simulink model "EjemploClient"  (Simulink 8.1)
settings: Solver=ode3  StartTime=0.0  StopTime=inf  FixedStep=0.01  RelTol=1e-3
libraries: aerolibanimutils x1
settings Model: Creator=Usuario  LastModifiedBy=emanuel
settings OptimizationCC: SimCompilerOptimization=On

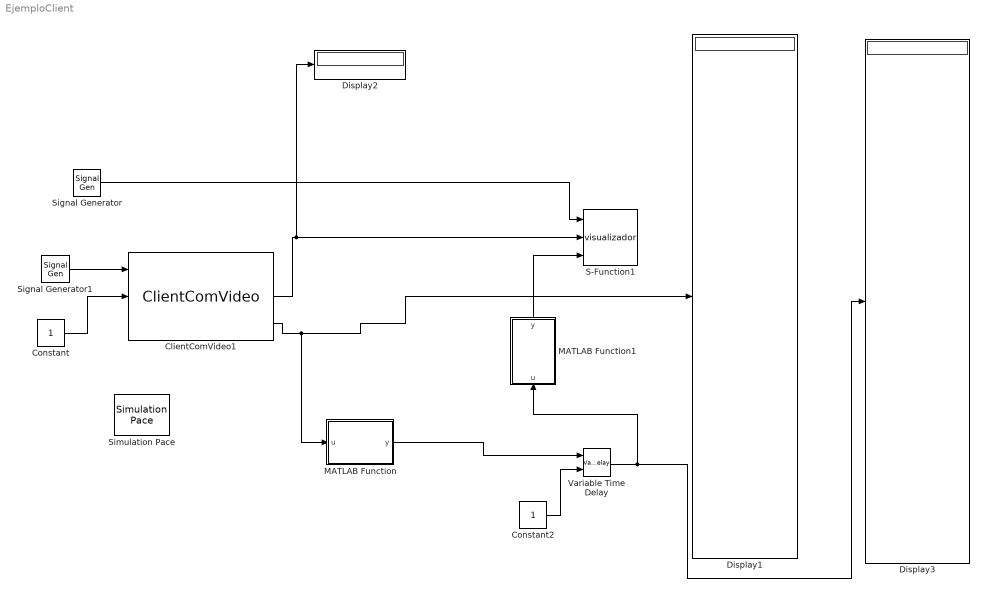
== system EjemploClient ==
  ClientComVideo1 : S-Function  FunctionName=ClientComVideo  EnableBusSupport=off
      mask Display:
      | patch([0 4. 4 0],[0.02 0.02 0.98 0.98],0.9*[123 193 255]/255)
      | patch([0 4 4 0],[0.1 0.1 0.9 0.9],[123 193 255]/255)
      | patch([1.5 2.5 2.5 2.3 2.3 1.7 1.7 1.5],[0 0 1 1 1.2 1.2 1 1],[130 130 130]/255)
      | patch([1.3 2.7 2.7 1.3],[1.2 1.2 2.9 2.9],0.85*[130 130 130]/255)
      | patch([1.4 2.6 2.6 1.4],[1.3 1.3 2.8 2.8],[123 193 255]/255)
      | patch([1.5 2.5 2.5 1.5],[1.4 1.4 2.7 2.7],0.85*[130 130 130]/255)
      | patch([1.9 2.1 2.1 1.9],[1.8 1.8 2.1 2.1],[123 193 255]/255)
      | color('red')
      | port_label('input',1,'clock')
      | port_label('input',2,'sizeSend')
      | port_label('input',3,'dataSend')
      | port_label('output',1,'stateChannel')
      | port_label('output',2,'sizeMustBeRecv')
      | port_label('output',3,'dataRecv')
  Constant : Constant  OutDataTypeStr=uint32
  Constant2 : Constant  OutDataTypeStr=double
  Display1 : Display
  Display2 : Display
  Display3 : Display
  MATLAB Function : MATLAB Function  TreatAsAtomicUnit=on
  MATLAB Function1 : MATLAB Function  TreatAsAtomicUnit=on
  S-Function1 : S-Function  FunctionName=visualizador  Parameters=1  EnableBusSupport=off
  Signal Generator : SignalGenerator  WaveForm=square  Frequency=20
  Signal Generator1 : SignalGenerator  WaveForm=square  Frequency=20
  Simulation Pace : aerolibanimutils/Simulation Pace  SimulationPace=1  SleepMode=MATLAB Thread  OutputPaceError=off  SampleTime=-1
      settings: AttributesFormatString=%<SimulationPace> sec/sec
  Variable Time Delay : VariableTransportDelay  MaximumDelay=10
  wires:
  Signal Generator/1 -> S-Function1/1
  Signal Generator1/1 -> ClientComVideo1/1
  Constant/1 -> ClientComVideo1/2
  ClientComVideo1/2 -> S-Function1/2, Display2/1
  ClientComVideo1/3 -> MATLAB Function/1(u), Display1/1
  Constant2/1 -> Variable Time Delay/2
  MATLAB Function/1(y) -> Variable Time Delay/1
  Variable Time Delay/1 -> Display3/1, MATLAB Function1/1(u)
  MATLAB Function1/1(y) -> S-Function1/3

== matlab function MATLAB Function1 ==
  data: u input double; y output double
function y = fcn(u)
%#codegen

y = uint8([u;zeros(60000-length(u),1)]);

== matlab function MATLAB Function ==
  data: u input double; y output double
function y = fcn(u)
%#codegen

y = double(u(1:5000));
